simulink model "Delay_Margin"  (R2024a)
settings: Solver=VariableStepAuto  StartTime=0.0  StopTime=10.0  MaxStep=0.01  RelTol=1e-3
values from neighbouring files (symbols this model uses):
  C = C_V{C_idx}    [Run.m]
  delay = delay_V{d_idx}    [Run.m]
  G = 1/(s^2 + 0.5*s + 1)    [Run.m]
settings Model: Creator=berto  LastModifiedBy=berto

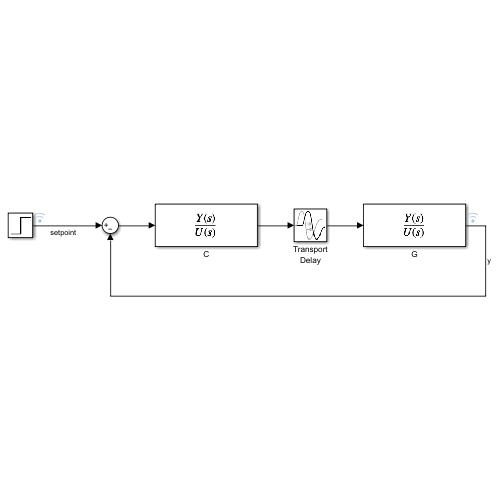
[thumbnail: Simulink's stored preview of the top-level diagram]
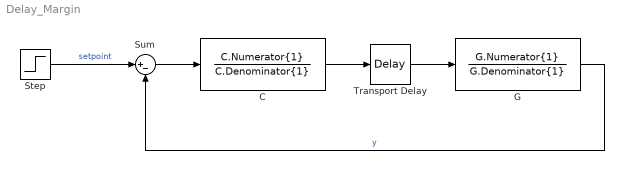
== system Delay_Margin ==
  C : TransferFcn  Numerator=C.Numerator{1}  Denominator=C.Denominator{1}
  G : TransferFcn  Numerator=G.Numerator{1}  Denominator=G.Denominator{1}
  Step : Step  SampleTime=0
  Sum : Sum  Inputs=|+-
  Transport Delay : TransportDelay  DelayTime=delay
  wires:
  C/1 -> Transport Delay/1
  Transport Delay/1 -> G/1
  Sum/1 -> C/1
  G/1 -> Sum/2  "y"
  Step/1 -> Sum/1  "setpoint"
